simulink model "boost_control"  (R2024b)
settings: Solver=VariableStepAuto  StartTime=0.0  StopTime=Tend  RelTol=1e-3
InitFcn:
  | %% Gerador
  | K_e = 5.4e-3; % Relação FEM/rotacao
  | p = 5; % Numero de pares de pólos
  | R_ger = 1.94; % mOhm - Conferir unidade no simulink
  | L_ger = 77; % uH - conferir unidade no simulink
  | f_min = 1800*p/60;
  | f_max = 8400*p/60;
  | 
  | %% Retificador trifásico
  | V_fwd = 1.46/2; % em Volts e I_fwd = 150A
  | R_on = (1.46-1.13)/(150 - 50); % Ohm - on resistance
  | G_off = 100/1200; % uS - off Conductance
  | 
  | %% Capacitores
  | C_in = 12; % mF - Conferir unidade no simulink
  | C_in_esr = 29; % mOhm
  | C_out = 12; % mF - Conferir unidade no simulink
  | C_out_esr = 29; % mOhm
  | 
  | %% Indutores
  | L = 80; % mH - Conferir unidade no simulink
  | R_L_min = 0.1; % mOhm
  | R_L_max = 100; % mOhm
  | R_L = (R_L_min + R_L_max)/2; % mOhm - Conferir unidade no simulink
  | 
  | %% PWM frequency
  | f_pwm = 10e3;
  | T_pwm = 1/f_pwm;
values from neighbouring files (symbols this model uses):
  Ts = 0.001    [boost_data.mat]    (also in teste_ukf.m = 1e-05; wynda_demo.m)
libraries: nesl_utility x1
settings Model: Creator=eric  LastModifiedBy=eric

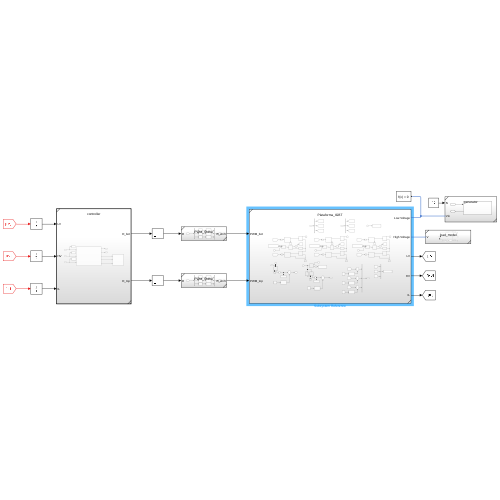
[thumbnail: Simulink's stored preview of the top-level diagram]
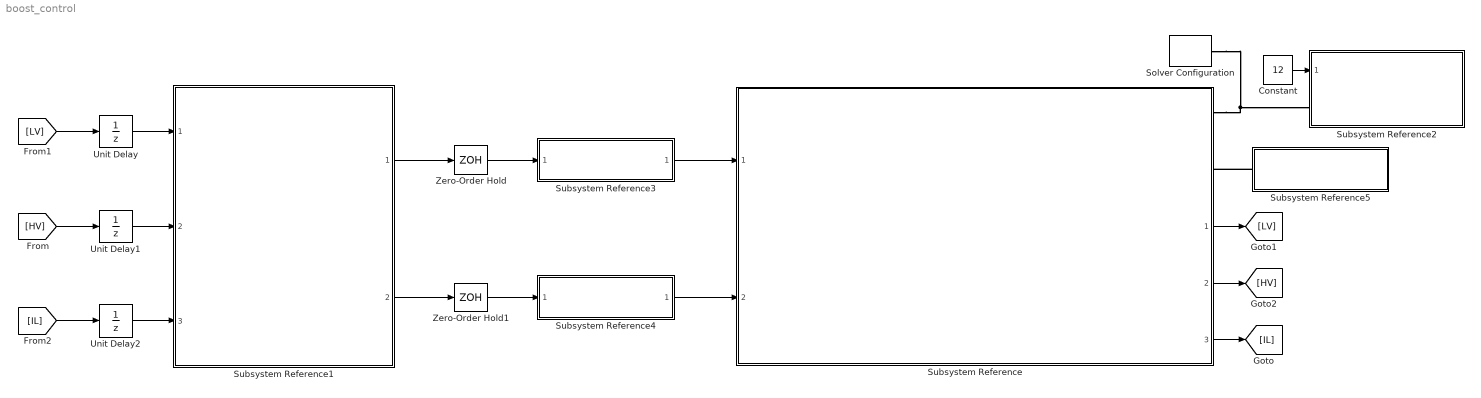
== system boost_control ==
  Constant : Constant  Value=12
  Solver Configuration : nesl_utility/Solver Configuration  PhysicalDomain=network_engine_domain  SubClassName=solver  LeftPortType=input  RightPortType=generic  Tones=[]  Harmonics=[]  SimulateNoise=off  Profile=off  UseLocalSampling=off  EnableSwitchedLinearOptims=on  FrequencyDomain=off  UseCCode=off  RelTol=0.001  AbsTol=0.001  MinStep=1e-09  ToWorkspace=off  RevertToSquareIcSolve=off  NumHomotopyIterations=100  PhasorMode=off  PhasorModeNumHarmonics=1  ConsistencySolver=NEWTON_XTOL_AFTER_FTOL  IndexReductionMethod=DerivativeReplacement  DoDC=off  ResidualTolerance=1e-09  ConsistencyTolSource=GLOBAL  ConsistencyAbsTol=0.001  ConsistencyRelTol=0.001  ConsistencyTolFactor=0.001  UseLocalSolver=off  LocalSolverChoice=NE_BACKWARD_EULER_ADVANCER  ResolveIndetEquations=on  FunctionEvalNumThread=1  LocalSolverSampleTime=0.001  DoFixedCost=off  MaxNonlinIter=3  MaxModeIter=2  ComputeImpulses=off  ImpulseIterations=2  LinearAlgebra=auto  LinearAlgebraNumThread=0  EquationFormulation=NE_TIME_EF  DelaysMemoryBudget=1024  AutomaticFiltering=on  FilteringTimeConstant=0.001  PartitionStorageMethod=AS_NEEDED  PartitionMemoryBudget=1024  PartitionMethod=ROBUST  MultibodyUseLocalSolver=off  MultibodyLocalSolverChoice=ODE1  MultibodyLocalSolverSampleTime=0.001
  Subsystem Reference : Subsystem  ReferencedSubsystem=Plataforma_IGBT
      settings: PortSchema="{\"entries\":[{\"content\":{\"sides\":[{\"content\":{\"connectorIds\":[\"In1\",\"In2\"]},\"type\":\"ConnectorPlacement.EquallySpacedRectSide\",\"uuid\":\"00713e95-3d7f-4851-838e-0146fde832ba\"},{\"content\":{\"connectorIds\":[\"LConn1\",\"LConn2\",\"Out1\",\"Out2\",\"Out3\"],\"side\":\"RIGHT\"},\"type\":\"ConnectorPlacement.EquallySpacedRectSide\",\"uuid\":\"8ae80668-bcf9-4189-9ae2-c64fbf014b23\"},{\"content\":{\"side\":\"TOP\"},\"type\":\"ConnectorPlacement.EquallySpacedRectSide\",\"uuid\":\"9387a63e-f699-459d-b536-bb96666c1de5\"}]},\"type\":\"ConnectorPlacement.EquallySpacedConnector\",\"uuid\":\"4db73444-77cb-42b9-92d1-e0dc7dafcf57\"}],\"packageUris\":[\"http://schema.mathworks.com/mf0/Connector/R2020b\"],\"version\":\"1.0\"}"
  Subsystem Reference1 : Subsystem  TreatAsAtomicUnit=on  SystemSampleTime=Ts  ReferencedSubsystem=controller
  Subsystem Reference2 : Subsystem  ReferencedSubsystem=generator
  Subsystem Reference3 : Subsystem  ReferencedSubsystem=PWM_Shifter
  Subsystem Reference4 : Subsystem  ReferencedSubsystem=PWM_Shifter
  Subsystem Reference5 : Subsystem  ReferencedSubsystem=load_model
  Unit Delay : UnitDelay  SampleTime=-1  HasFrameUpgradeWarning=on
  Unit Delay1 : UnitDelay  SampleTime=-1  HasFrameUpgradeWarning=on
  Unit Delay2 : UnitDelay  SampleTime=-1  HasFrameUpgradeWarning=on
  Zero-Order Hold : ZeroOrderHold  SampleTime=T_pwm
  Zero-Order Hold1 : ZeroOrderHold  SampleTime=T_pwm
  wires:
  Constant/1 -> Subsystem Reference2/1
  Subsystem Reference/3 -> [IL]
  Subsystem Reference/1 -> [LV]
  Subsystem Reference/2 -> [HV]
  Subsystem Reference1/2 -> Zero-Order Hold1/1
  Subsystem Reference1/1 -> Zero-Order Hold/1
  Zero-Order Hold1/1 -> Subsystem Reference4/1
  Zero-Order Hold/1 -> Subsystem Reference3/1
  Subsystem Reference4/1 -> Subsystem Reference/2
  Subsystem Reference3/1 -> Subsystem Reference/1
  [LV] -> Unit Delay/1
  [HV] -> Unit Delay1/1
  [IL] -> Unit Delay2/1
  Unit Delay/1 -> Subsystem Reference1/1
  Unit Delay1/1 -> Subsystem Reference1/2
  Unit Delay2/1 -> Subsystem Reference1/3
  connections:
  Subsystem Reference/LConn1 -- Solver Configuration/RConn1 -- Subsystem Reference2/LConn1
  Subsystem Reference5/LConn1 -- Subsystem Reference/LConn2
